simulink model "untitled - Copy"  (R2023b)
settings: Solver=VariableStepAuto  StartTime=0.0  StopTime=10  RelTol=1e-3
settings Model: Creator=nurbi  LastModifiedBy=nurbi

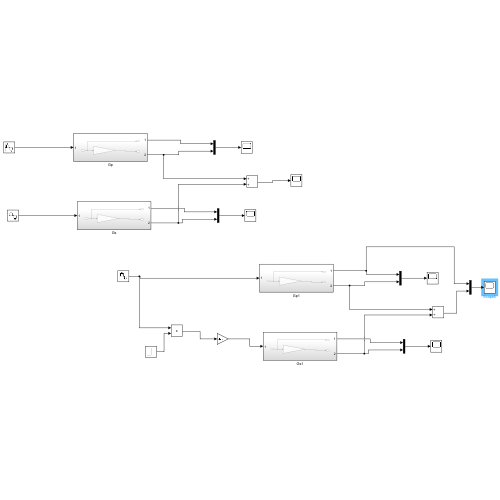
[thumbnail: Simulink's stored preview of the top-level diagram]
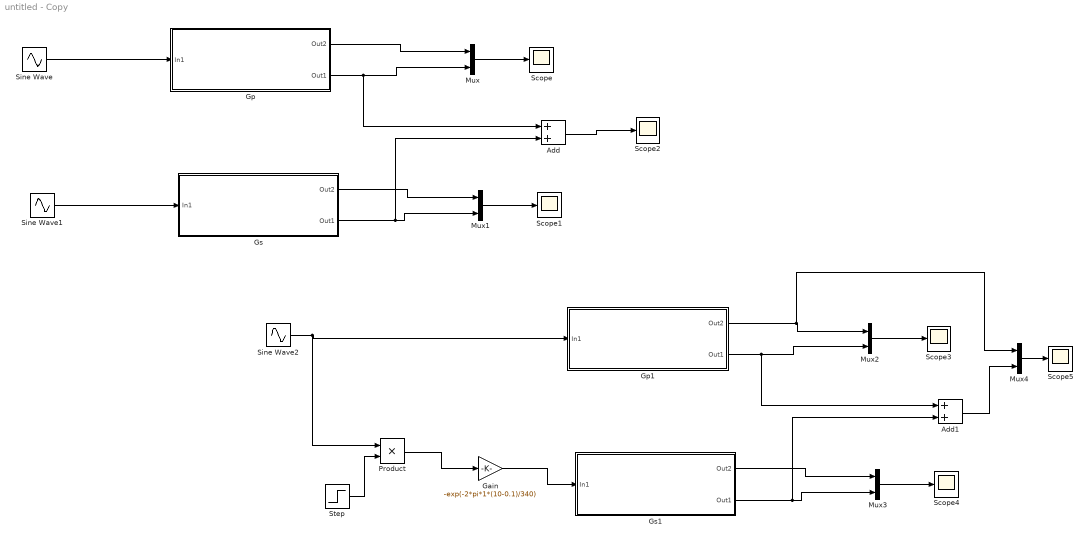
== system untitled - Copy ==
  Add : Sum
  Add1 : Sum
  Gain : Gain  Gain=-exp(-2*pi*1*(10-0.1)/340)
  Gp : Subsystem
  Gp1 : Subsystem
  Gs : Subsystem
  Gs1 : Subsystem
  Mux{,1..4} (5 alike) : Mux  Inputs=2
  Product : Product
  Scope{,1..5} (6 alike) : Scope
  Sine Wave : Sin  Frequency=2*pi*10  SampleTime=0.001
  Sine Wave1 : Sin  Frequency=2*pi*1  SampleTime=0.001
  Sine Wave2 : Sin  Frequency=2*pi*10  SampleTime=0.001
  Step : Step  Time=5  SampleTime=0
  wires:
  Mux/1 -> Scope/1
  Sine Wave/1 -> Gp/1(In1)
  Gp/1(Out2) -> Mux/1
  Mux1/1 -> Scope1/1
  Sine Wave1/1 -> Gs/1(In1)
  Gs/1(Out2) -> Mux1/1
  Gs/2(Out1) -> Add/2, Mux1/2
  Add/1 -> Scope2/1
  Gp/2(Out1) -> Add/1, Mux/2
  Gp1/2(Out1) -> Add1/1, Mux2/2
  Gs1/1(Out2) -> Mux3/1
  Mux3/1 -> Scope4/1
  Gs1/2(Out1) -> Add1/2, Mux3/2
  Mux2/1 -> Scope3/1
  Sine Wave2/1 -> Product/1, Gp1/1(In1)
  Gain/1 -> Gs1/1(In1)
  Mux4/1 -> Scope5/1
  Add1/1 -> Mux4/2
  Gp1/1(Out2) -> Mux4/1, Mux2/1
  Step/1 -> Product/2
  Product/1 -> Gain/1

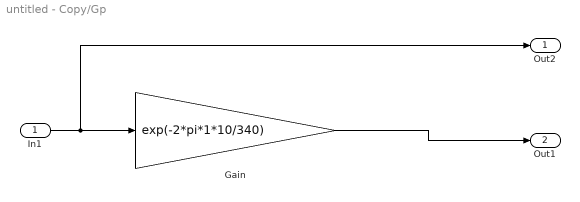
== system untitled - Copy/Gp ==
  In1 : Inport
  Gain : Gain  Gain=exp(-2*pi*1*10/340)
  Out2 : Outport
  Out1 : Outport  Port=2
  wires:
  In1/1 -> Out2/1, Gain/1
  Gain/1 -> Out1/1

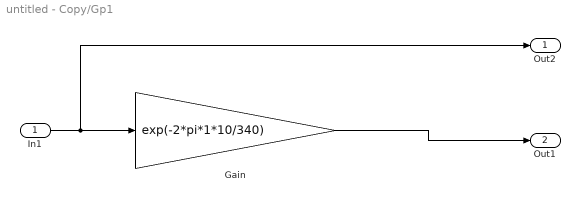
== system untitled - Copy/Gp1 ==
  In1 : Inport
  Gain : Gain  Gain=exp(-2*pi*1*10/340)
  Out2 : Outport
  Out1 : Outport  Port=2
  wires:
  In1/1 -> Out2/1, Gain/1
  Gain/1 -> Out1/1

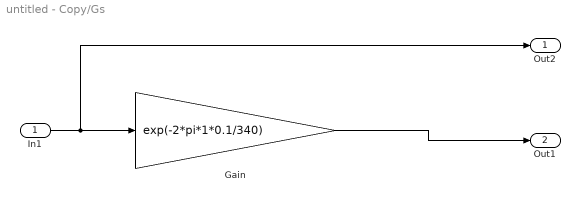
== system untitled - Copy/Gs ==
  In1 : Inport
  Gain : Gain  Gain=exp(-2*pi*1*0.1/340)
  Out2 : Outport
  Out1 : Outport  Port=2
  wires:
  In1/1 -> Out2/1, Gain/1
  Gain/1 -> Out1/1

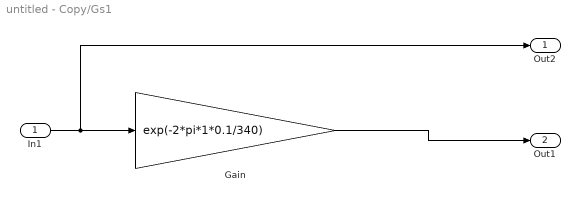
== system untitled - Copy/Gs1 ==
  In1 : Inport
  Gain : Gain  Gain=exp(-2*pi*1*0.1/340)
  Out2 : Outport
  Out1 : Outport  Port=2
  wires:
  In1/1 -> Out2/1, Gain/1
  Gain/1 -> Out1/1
